simulink model "sl_ztorqueFreefall"  (R2014a)
settings: Solver=ode45  StartTime=0.0  StopTime=2.5  RelTol=1e-3
values from neighbouring files (symbols this model uses):
  q_in = [ 0 0 0 0 0 0]'    [Project3_Dockter.m]    (also in Project3sampleCode.m)
libraries: roblocks x2
settings Model: ExtModeTrigMode=oneshot  ExtModeArmWhenConnect=off  Creator=pic  LastModifiedBy=MRDLAB
settings DataIOCC: LimitDataPoints=off  SignalLoggingSaveFormat=ModelDataLogs  SignalLogging=off  ReturnWorkspaceOutputs=on
settings OptimizationCC: BlockReduction=off  BooleanDataType=off  ExpressionDepthLimit=2147483647  InitFltsAndDblsToZero=on
settings DebuggingCC: SaveWithParameterizedLinksMsg=none  UnderspecifiedInitializationDetection=Classic  SignalResolutionControl=TryResolveAllWithWarning  SolverPrmCheckMsg=none  MultiTaskDSMMsg=warning  MultiTaskCondExecSysMsg=none  FcnCallInpInsideContextMsg=UseLocalSettings  StateNameClashWarn=warning
settings HardwareCC: TargetUnknown=on
settings RTWCC: IncludeERTFirstTime=on
settings GRTTargetCC: ModelReferenceCompliant=off  ParMdlRefBuildCompliant=off  CompOptLevelCompliant=off  CombineOutputUpdateFcns=off  MatFileLogging=off  GRTInterface=on

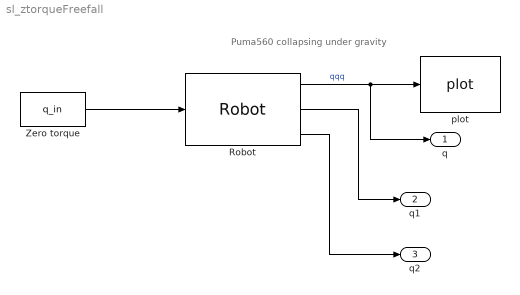
== system sl_ztorqueFreefall ==
  note: Puma560 collapsing under gravity
  Robot : roblocks/Dynamics/Robot  robot=myRobot  q0=q0
      link override Integrator: InitialCondition=qd0
  Zero torque : Constant  Value=q_in
  plot : roblocks/Robot Graphics/plot  robot=p560  fps=25  holdplot=on
  q : Outport
  q1 : Outport  Port=2
  q2 : Outport  Port=3
  wires:
  Robot/1 -> plot/1, q/1  "qqq"
  Robot/3 -> q2/1
  Robot/2 -> q1/1
  Zero torque/1 -> Robot/1
